simulink model "sampleModel250"  (R2021b)
settings: Solver=VariableStepAuto  StartTime=0.0  StopTime=10.0  RelTol=1e-3
undefined symbols (not defined in the file or in its folder): DiscIntNeverNeededParam, Newton, Raphson
libraries: simulink x19, slpidlib x2
settings Model: Creator=user  LastModifiedBy=user

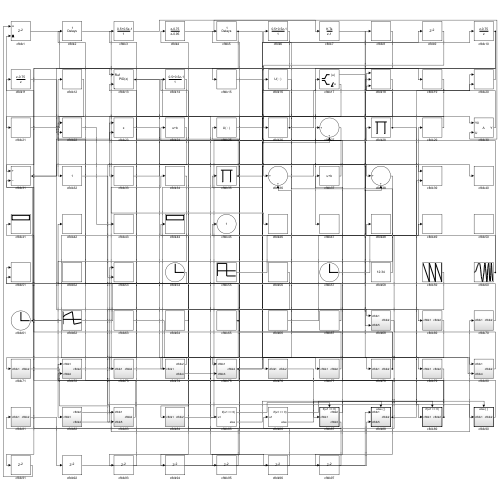
[thumbnail: Simulink's stored preview of the top-level diagram]
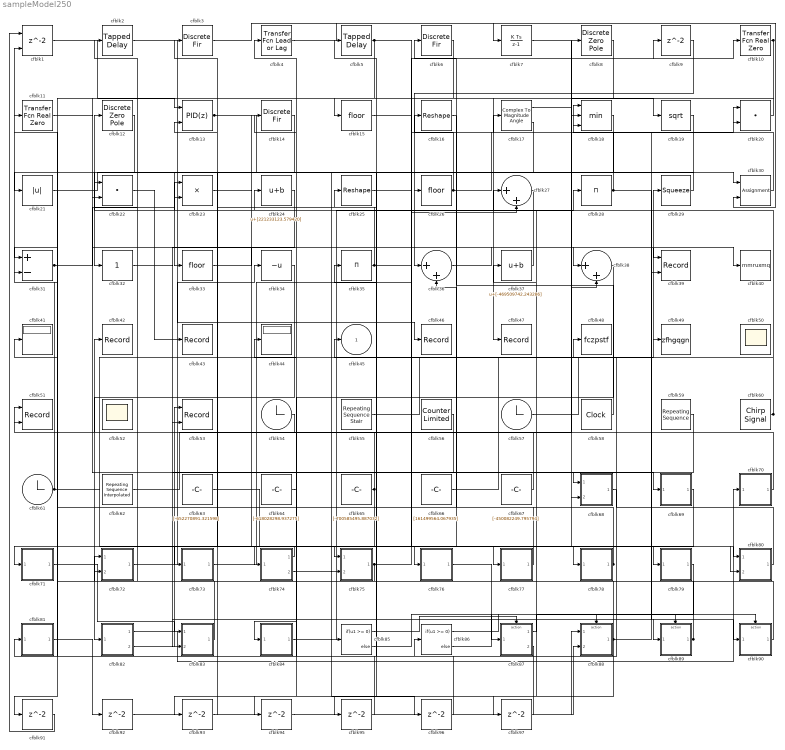
== system sampleModel250 ==
  cfblk1 : Delay  ShowEnablePort=on  SampleTime=1
      settings: InputPortMap=u0,e6
  cfblk10 : simulink/Discrete/Transfer Fcn Real Zero  ZeroZ=0.75  ICPrevInput=0.0  DoSatur=off
      settings: SourceProductBaseCode=SL
  cfblk11 : simulink/Discrete/Transfer Fcn Real Zero  ZeroZ=0.75  ICPrevInput=0.0  DoSatur=off
      settings: SourceProductBaseCode=SL
  cfblk12 : DiscreteZeroPole  Poles=[0 0.5]  Gain=1
  cfblk13 : slpidlib/PID Controller (2DOF)  Controller=PID  Form=Parallel  TimeDomain=Discrete-time  UseExternalTs=off  SampleTime=1  IntegratorMethod=Forward Euler  FilterMethod=Forward Euler  ControllerParametersSource=internal  P=1  I=1  D=0  UseFilter=on  N=100  b=1  c=1  TunerSelectOption=Transfer Function Based (PID Tuner App)  InitialConditionSource=internal  InitialConditionForIntegrator=0  InitialConditionForFilter=0  DifferentiatorICPrevScaledInput=0  ExternalReset=none  TrackingMode=off  Kt=1  LimitOutput=off  SatLimitsSource=internal  UpperSaturationLimit=inf  LowerSaturationLimit=-inf  LinearizeAsGain=off  AntiWindupMode=none  Kb=1  POutMin=[]  POutMax=[]  IOutMin=[]  IOutMax=[]  DOutMin=[]  DOutMax=[]  NOutMin=[]  NOutMax=[]  bOutMin=[]  bOutMax=[]  cOutMin=[]  cOutMax=[]  SumOutMin=[]  SumOutMax=[]  SaturationOutMin=[]  SaturationOutMax=[]  PParamMin=[]  PParamMax=[]  IParamMin=[]  IParamMax=[]  DParamMin=[]  DParamMax=[]  NParamMin=[]  NParamMax=[]  bParamMin=[]  bParamMax=[]  cParamMin=[]  cParamMax=[]  KbParamMin=[]  KbParamMax=[]  KtParamMin=[]  KtParamMax=[]  KbOutMin=[]  KbOutMax=[]  KtOutMin=[]  KtOutMax=[]  IntegratorOutMin=[]  IntegratorOutMax=[]  FilterOutMin=[]  FilterOutMax=[]  SumI1OutMin=[]  SumI1OutMax=[]  SumI2OutMin=[]  SumI2OutMax=[]  SumI3OutMin=[]  SumI3OutMax=[]  SumI4OutMin=[]  SumI4OutMax=[]  SumDOutMin=[]  SumDOutMax=[]  Sum1OutMin=[]  Sum1OutMax=[]  Sum2OutMin=[]  Sum2OutMax=[]  Sum3OutMin=[]  Sum3OutMax=[]  DifferentiatorOutMin=[]  DifferentiatorOutMax=[]  FilterDiffOutCoefMin=[]  FilterDiffOutCoefMax=[]  ReciprocalOutMin=[]  ReciprocalOutMax=[]  SumDenOutMin=[]  SumDenOutMax=[]  SumNumOutMin=[]  SumNumOutMax=[]  DivideOutMin=[]  DivideOutMax=[]  UdiffTsProdOutMin=[]  UdiffTsProdOutMax=[]  NTsProdOutMin=[]  NTsProdOutMax=[]  UintegralTsProdOutMin=[]  UintegralTsProdOutMax=[]  UngainTsProdOutMin=[]  UngainTsProdOutMax=[]  IntegratorContinuousStateAttributes=''  IntegratorStateMustResolveToSignalObject=off  IntegratorRTWStateStorageClass=Auto  FilterContinuousStateAttributes=''  FilterStateMustResolveToSignalObject=off  FilterRTWStateStorageClass=Auto  ParallelPVariant=InternalParameters  IdealPVariant=Disabled  IVariant=InternalParameters  DVariant=InternalParameters  bVariant=InternalParameters  cVariant=InternalParameters  IntegratorVariant=Discrete  SatVariant=Disabled  AWVariant=Passthrough  PCopyVariant=Disabled  TRVariant=Disabled  FdbkBlocksVariant=Forward  IdealPFdbkVariant=Disabled  SatFdbkVariant=Disabled  DerivativeFilterVariant=ForwardEulerFilter  NVariant=InternalParameters  NCopyVariant=Disabled  FilterICVariant=InternalICsFilter  IntegratorICVariant=InternalICs  ExternalResetVariant=Disabled  TRSumVariant=Passthrough  SumFdbkVariant=Disabled  SumVariant=Sum_PID  TsampFilterVariant=InternalTs  TsampNgainVariant=Passthrough  TsampIntegralVariant=Passthrough  ExternalSaturationOutDataTypeStr=Inherit: Same as second input
      settings: SourceProductBaseCode=SL
  cfblk14 : DiscreteFir  SampleTime=1
  cfblk15 : Rounding
  cfblk16 : Reshape
  cfblk17 : ComplexToMagnitudeAngle
  cfblk18 : MinMax  Inputs=3
  cfblk19 : Sqrt  SaturateOnIntegerOverflow=on
  cfblk2 : simulink/Discrete/Tapped Delay  vinit=0.0  samptime=-1  NumDelays=1  DelayOrder=Oldest  includeCurrent=off
  cfblk20 : DotProduct  InputSameDT=on  OutDataTypeStr=Inherit: Inherit via internal rule
  cfblk21 : Abs
  cfblk22 : DotProduct  InputSameDT=on  OutDataTypeStr=Inherit: Inherit via internal rule
  cfblk23 : Product
  cfblk24 : Bias  Bias=[221233123.579420]
  cfblk25 : Reshape
  cfblk26 : Rounding
  cfblk27 : Sum  Inputs=|++
  cfblk28 : Product  Inputs=*
  cfblk29 : Squeeze
  cfblk3 : DiscreteFir  SampleTime=1
  cfblk30 : Assignment  DiagnosticForDimensions=Warning  IndexOptions=Index vector (dialog)  Indices=1  OutputSizes=1
  cfblk31 : Sum  Inputs=+-
  cfblk32 : simulink/Math Operations/Slider Gain  gain=1  low=0  high=2
  cfblk33 : Rounding
  cfblk34 : UnaryMinus
  cfblk35 : Product  Inputs=*
  cfblk36 : Sum  Inputs=|++
  cfblk37 : Bias  Bias=[-469509742.243286]
  cfblk38 : Sum  Inputs=|++
  cfblk39 : Record  FileSettingsInternal="{\"entries\":[{\"content\":{\"excelSettings\":{\"content\":{},\"type\":\"Streamout.ExcelSettings\"}},\"type\":\"Streamout.FileSettingStorage\",\"uuid\":\"39295518-5782-4a04-9dda-65bbf2f7290d\"}],\"packageUris\":[\"http://schema.mathworks.com/mf0/streamout_blocks/R2020a\"],\"version\":\"1.0\"}"  Layout=[1 1]  SignalsInternal="{\"entries\":[{\"content\":{\"signals\":[{\"content\":{\"blockPath\":[\"sampleModel250/cfblk39\"],\"channel\":[],\"dimensions\":[1],\"domain\":\"sampleModel250/cfblk39\",\"lineColor\":\"#a2142f\",\"plots\":[1],\"port\":1,\"sid\":[\"\"],\"signalID\":10132,\"signalName\":\"cfblk33\"},\"type\":\"RecordBlkView.Signal\",\"uuid\":\"9efbc733-4780-4410-b863-ce1b8cd8a036\"},{\"content\":{\"blockPath\":[\"sampleModel250/cfblk39\"],\"channel\":[],\"dimensions\":[1],\"domain\":\"sampleModel250/cfblk39\",\"lineColor\":\"#139fff\",\"plots\":[1],\"port\":2,\"sid\":[\"\"],\"signalID\":10136,\"signalName\":\"cfblk61\"},\"type\":\"RecordBlkView.Signal\",\"uuid\":\"712e342f-030a-4a03-987d-c30699e0cda9\"}]},\"type\":\"RecordBlkView.InputSignals\",\"uuid\":\"45709923-ac2f-4e8a-b5ce-1ea2a88c9728\"}],\"packageUris\":[\"http://schema.mathworks.com/mf0/streamout_blocks/R2020a\"],\"version\":\"1.0\"}"  VisualizationBindings="{\"xyplotplugin\":{\"info\":[{\"series\":[{\"bindingParametersList\":[{\"parameter\":\"X-Axis\",\"signalID\":10132,\"signalName\":\"cfblk33\"},{\"parameter\":\"Y-Axis\",\"signalID\":10136,\"signalName\":\"cfblk61\"}],\"seriesID\":11867}],\"subplotID\":1}]}}"  CompatibilityTag=XY
  cfblk4 : simulink/Discrete/Transfer Fcn Lead or Lag  PoleZ=0.95  ZeroZ=0.75  ICPrevOutput=0.0  ICPrevInput=0.0  DoSatur=off
      settings: SourceProductBaseCode=SL
  cfblk40 : ToWorkspace  VariableName=mmruxmq  SaveFormat=Timeseries  SampleTime=-1
  cfblk41 : Display
  cfblk42 : Record  FileSettingsInternal="{\"entries\":[{\"content\":{\"excelSettings\":{\"content\":{},\"type\":\"Streamout.ExcelSettings\"}},\"type\":\"Streamout.FileSettingStorage\",\"uuid\":\"cb9cef44-850f-46f8-9e62-a5d9019da7f8\"}],\"packageUris\":[\"http://schema.mathworks.com/mf0/streamout_blocks/R2020a\"],\"version\":\"1.0\"}"  SignalsInternal="{\"entries\":[{\"content\":{\"signals\":[{\"content\":{\"blockPath\":[\"sampleModel250/cfblk42\"],\"channel\":[],\"dimensions\":[1],\"domain\":\"sampleModel250/cfblk42\",\"lineColor\":\"#0072bd\",\"plots\":[1],\"port\":1,\"sid\":[\"\"],\"signalID\":10168,\"signalName\":\"cfblk67\"},\"type\":\"RecordBlkView.Signal\",\"uuid\":\"09506a4d-d469-40bf-9df4-0557f256c8fa\"}]},\"type\":\"RecordBlkView.InputSignals\",\"uuid\":\"d07d11bf-0a13-4a29-ba0c-274f99fcec3c\"}],\"packageUris\":[\"http://schema.mathworks.com/mf0/streamout_blocks/R2020a\"],\"version\":\"1.0\"}"  VisualizationBindings="{\"sparklinesplugin\":{\"info\":[{\"bindingParametersList\":[],\"subplotID\":1}]}}"
  cfblk43 : Record  FileSettingsInternal="{\"entries\":[{\"content\":{\"excelSettings\":{\"content\":{},\"type\":\"Streamout.ExcelSettings\"}},\"type\":\"Streamout.FileSettingStorage\",\"uuid\":\"24f78354-d28b-420c-ba3f-fe416d6032e0\"}],\"packageUris\":[\"http://schema.mathworks.com/mf0/streamout_blocks/R2020a\"],\"version\":\"1.0\"}"  SignalsInternal="{\"entries\":[{\"content\":{\"signals\":[{\"content\":{\"blockPath\":[\"sampleModel250/cfblk43\"],\"channel\":[],\"dimensions\":[1],\"domain\":\"sampleModel250/cfblk43\",\"lineColor\":\"#139fff\",\"plots\":[1],\"port\":1,\"sid\":[\"\"],\"signalID\":10140,\"signalName\":\"cfblk22\"},\"type\":\"RecordBlkView.Signal\",\"uuid\":\"c1a6c549-0a82-4f1d-8783-18ee6ca6e206\"}]},\"type\":\"RecordBlkView.InputSignals\",\"uuid\":\"009778dc-f500-4119-a494-20fbbf5a50bc\"}],\"packageUris\":[\"http://schema.mathworks.com/mf0/streamout_blocks/R2020a\"],\"version\":\"1.0\"}"  VisualizationBindings="{\"sparklinesplugin\":{\"info\":[{\"bindingParametersList\":[],\"subplotID\":1}]}}"
  cfblk44 : Display
  cfblk46 : Record  FileSettingsInternal="{\"entries\":[{\"content\":{\"excelSettings\":{\"content\":{},\"type\":\"Streamout.ExcelSettings\"}},\"type\":\"Streamout.FileSettingStorage\",\"uuid\":\"d34b3b38-d37b-44bf-a1ca-0d6c239076fa\"}],\"packageUris\":[\"http://schema.mathworks.com/mf0/streamout_blocks/R2020a\"],\"version\":\"1.0\"}"  SignalsInternal="{\"entries\":[{\"content\":{\"signals\":[{\"content\":{\"blockPath\":[\"sampleModel250/cfblk46\"],\"channel\":[],\"dimensions\":[1],\"domain\":\"sampleModel250/cfblk46\",\"lineColor\":\"#ff6929\",\"plots\":[1],\"port\":1,\"sid\":[\"\"],\"signalID\":10144,\"signalName\":\"cfblk2\"},\"type\":\"RecordBlkView.Signal\",\"uuid\":\"5d42b0a2-1079-46c0-88f1-f1e7f1e913a3\"}]},\"type\":\"RecordBlkView.InputSignals\",\"uuid\":\"de118d10-f6e7-4dc8-9a86-7f08f8c21061\"}],\"packageUris\":[\"http://schema.mathworks.com/mf0/streamout_blocks/R2020a\"],\"version\":\"1.0\"}"  VisualizationBindings="{\"sparklinesplugin\":{\"info\":[{\"bindingParametersList\":[],\"subplotID\":1}]}}"
  cfblk47 : Record  FileSettingsInternal="{\"entries\":[{\"content\":{\"excelSettings\":{\"content\":{},\"type\":\"Streamout.ExcelSettings\"}},\"type\":\"Streamout.FileSettingStorage\",\"uuid\":\"d3a56f26-8ac3-44b7-90be-3d39ad570db3\"}],\"packageUris\":[\"http://schema.mathworks.com/mf0/streamout_blocks/R2020a\"],\"version\":\"1.0\"}"  SignalsInternal="{\"entries\":[{\"content\":{\"signals\":[{\"content\":{\"blockPath\":[\"sampleModel250/cfblk47\"],\"channel\":[],\"dimensions\":[1],\"domain\":\"sampleModel250/cfblk47\",\"lineColor\":\"#b746ff\",\"plots\":[1],\"port\":1,\"sid\":[\"\"],\"signalID\":10148,\"signalName\":\"cfblk10\"},\"type\":\"RecordBlkView.Signal\",\"uuid\":\"91dbde0a-49a0-40fd-acb2-10672f723bb8\"}]},\"type\":\"RecordBlkView.InputSignals\",\"uuid\":\"eb8da581-21b2-4b6f-8b31-33cd9e31a0d9\"}],\"packageUris\":[\"http://schema.mathworks.com/mf0/streamout_blocks/R2020a\"],\"version\":\"1.0\"}"  VisualizationBindings="{\"sparklinesplugin\":{\"info\":[{\"bindingParametersList\":[],\"subplotID\":1}]}}"
  cfblk48 : ToWorkspace  VariableName=fczpstf  SaveFormat=Timeseries  SampleTime=-1
  cfblk49 : ToWorkspace  VariableName=zfhgqgn  SaveFormat=Timeseries  SampleTime=-1
  cfblk5 : simulink/Discrete/Tapped Delay  vinit=0.0  samptime=-1  NumDelays=1  DelayOrder=Oldest  includeCurrent=off
  cfblk50 : Scope
      settings: Floating=on
  cfblk51 : Record  FileSettingsInternal="{\"entries\":[{\"content\":{\"excelSettings\":{\"content\":{},\"type\":\"Streamout.ExcelSettings\"}},\"type\":\"Streamout.FileSettingStorage\",\"uuid\":\"966ac46e-7d6c-426f-9254-bf47747501fd\"}],\"packageUris\":[\"http://schema.mathworks.com/mf0/streamout_blocks/R2020a\"],\"version\":\"1.0\"}"  Layout=[1 1]  SignalsInternal="{\"entries\":[{\"content\":{\"signals\":[{\"content\":{\"blockPath\":[\"sampleModel250/cfblk51\"],\"channel\":[],\"dimensions\":[1],\"domain\":\"sampleModel250/cfblk51\",\"lineColor\":\"#a2142f\",\"plots\":[1],\"port\":1,\"sid\":[\"\"],\"signalID\":10152,\"signalName\":\"cfblk70\"},\"type\":\"RecordBlkView.Signal\",\"uuid\":\"bcb4d5db-4b3e-4679-994d-15607dbef0df\"},{\"content\":{\"blockPath\":[\"sampleModel250/cfblk51\"],\"channel\":[],\"dimensions\":[1],\"domain\":\"sampleModel250/cfblk51\",\"lineColor\":\"#139fff\",\"plots\":[1],\"port\":2,\"sid\":[\"\"],\"signalID\":10156,\"signalName\":\"cfblk54\"},\"type\":\"RecordBlkView.Signal\",\"uuid\":\"a7bcb3c4-7ca9-4d29-a0f0-397de417030a\"}]},\"type\":\"RecordBlkView.InputSignals\",\"uuid\":\"211dfadc-f85f-49df-8759-cd0fd8e255c0\"}],\"packageUris\":[\"http://schema.mathworks.com/mf0/streamout_blocks/R2020a\"],\"version\":\"1.0\"}"  VisualizationBindings="{\"xyplotplugin\":{\"info\":[{\"series\":[{\"bindingParametersList\":[{\"parameter\":\"X-Axis\",\"signalID\":10152,\"signalName\":\"cfblk70\"},{\"parameter\":\"Y-Axis\",\"signalID\":10156,\"signalName\":\"cfblk54\"}],\"seriesID\":32821}],\"subplotID\":1}]}}"  CompatibilityTag=XY
  cfblk52 : Scope
      settings: Floating=on
  cfblk53 : Record  FileSettingsInternal="{\"entries\":[{\"content\":{\"excelSettings\":{\"content\":{},\"type\":\"Streamout.ExcelSettings\"}},\"type\":\"Streamout.FileSettingStorage\",\"uuid\":\"99a0b977-80ef-4c26-b42d-8fc2480f20f4\"}],\"packageUris\":[\"http://schema.mathworks.com/mf0/streamout_blocks/R2020a\"],\"version\":\"1.0\"}"  Layout=[1 1]  SignalsInternal="{\"entries\":[{\"content\":{\"signals\":[{\"content\":{\"blockPath\":[\"sampleModel250/cfblk53\"],\"channel\":[],\"dimensions\":[1],\"domain\":\"sampleModel250/cfblk53\",\"lineColor\":\"#a2142f\",\"plots\":[1],\"port\":1,\"sid\":[\"\"],\"signalID\":10160,\"signalName\":\"cfblk82:2\"},\"type\":\"RecordBlkView.Signal\",\"uuid\":\"1e65bc9d-8603-4a2e-9d1d-7b919e3292a0\"},{\"content\":{\"blockPath\":[\"sampleModel250/cfblk53\"],\"channel\":[],\"dimensions\":[1],\"domain\":\"sampleModel250/cfblk53\",\"lineColor\":\"#139fff\",\"plots\":[1],\"port\":2,\"sid\":[\"\"],\"signalID\":10164,\"signalName\":\"cfblk24\"},\"type\":\"RecordBlkView.Signal\",\"uuid\":\"1291a606-ac13-4bc6-a3d7-eb7377e9d85e\"}]},\"type\":\"RecordBlkView.InputSignals\",\"uuid\":\"aee4432a-cd5b-40e7-8b3a-2ad3dc5d4c9c\"}],\"packageUris\":[\"http://schema.mathworks.com/mf0/streamout_blocks/R2020a\"],\"version\":\"1.0\"}"  VisualizationBindings="{\"xyplotplugin\":{\"info\":[{\"series\":[{\"bindingParametersList\":[{\"parameter\":\"X-Axis\",\"signalID\":10160,\"signalName\":\"cfblk82:2\"},{\"parameter\":\"Y-Axis\",\"signalID\":10164,\"signalName\":\"cfblk24\"}],\"seriesID\":43266}],\"subplotID\":1}]}}"  CompatibilityTag=XY
  cfblk54 : Clock
  cfblk55 : simulink/Sources/Repeating Sequence Stair  OutValues=[579601024.933068, -400366002.756727]  tsamp=-1  OutMin=[]  OutMax=[]  OutDataTypeStr=double  OutputDataTypeScalingMode=double  OutDataType=fixdt(0,8)  ConRadixGroup=Best Precision: Vector-wise  OutScaling=2^-12
  cfblk56 : simulink/Sources/Counter Limited  uplimit=[457.000000]  tsamp=-1
  cfblk57 : Clock
  cfblk58 : DigitalClock
  cfblk59 : simulink/Sources/Repeating Sequence  rep_seq_t=[0 2]  rep_seq_y=[908061452.879816, -156366852.799595]
  cfblk6 : DiscreteFir  SampleTime=1
  cfblk60 : simulink/Sources/Chirp Signal  f1=[877541552.872540]  T=[-602399763.720180]  f2=[-816781693.848202]
  cfblk61 : Clock
  cfblk62 : simulink/Sources/Repeating Sequence Interpolated  OutValues=[233966107.012773, 455224158.955072, 827697630.012159, -499442249.113524, -329990226.707010]  TimeValues=[0 0.1 0.5 0.6 1].'  LookUpMeth=Use Input Nearest  tsamp=0.01  OutMin=[]  OutMax=[]  OutDataTypeStr=double  OutputDataTypeScalingMode=double  OutDataType=fixdt(0,8)  OutScaling=2^-10
  cfblk63 : Constant  Value=[-652270891.321598]  SampleTime=1
  cfblk64 : Constant  Value=[-618028298.937275]  SampleTime=1
  cfblk65 : Constant  Value=[-700585495.887032]  SampleTime=1
  cfblk66 : Constant  Value=[161499564.067935]  SampleTime=1
  cfblk67 : Constant  Value=[-450082249.795794]  SampleTime=1
  cfblk68 : Subsystem
  cfblk69 : Subsystem
  cfblk7 : DiscreteIntegrator  ICPrevOutput=DiscIntNeverNeededParam  ICPrevScaledInput=DiscIntNeverNeededParam
  cfblk70 : Subsystem
  cfblk71 : Subsystem
  cfblk72 : Subsystem
  cfblk73 : Subsystem
  cfblk74 : Subsystem
  cfblk75 : Subsystem
  cfblk76 : Subsystem
  cfblk77 : Subsystem
  cfblk78 : Subsystem
  cfblk79 : Subsystem
  cfblk8 : DiscreteZeroPole  Poles=[0 0.5]  Gain=1
  cfblk80 : Subsystem
  cfblk81 : Subsystem
  cfblk82 : Subsystem
  cfblk83 : Subsystem
  cfblk84 : Subsystem
  cfblk85 : If  IfExpression=u1 >= 0  SampleTime=1
  cfblk86 : If  IfExpression=u1 >= 0  SampleTime=1
  cfblk87 : Subsystem  TreatAsAtomicUnit=on
  cfblk88 : Subsystem  TreatAsAtomicUnit=on
  cfblk89 : Subsystem  TreatAsAtomicUnit=on
  cfblk{9,91..97} (8 alike) : Delay  SampleTime=1
  cfblk90 : Subsystem  TreatAsAtomicUnit=on
  cfblk45 : Outport
  wires:
  cfblk2/1 -> cfblk46/1
  cfblk10/1 -> cfblk47/1, cfblk22/2
  cfblk72/1(cfblk2) -> cfblk34/1
  cfblk22/1 -> cfblk43/1
  cfblk9/1 -> cfblk36/1
  cfblk87/1(cfblk2) -> cfblk37/1
  cfblk68/1(cfblk2) -> cfblk86/1
  cfblk19/1 -> cfblk32/1
  cfblk82/1(cfblk2) -> cfblk70/1(cfblk1)
  cfblk29/1 -> cfblk26/1
  cfblk84/1(cfblk2) -> cfblk28/1
  cfblk37/1 -> cfblk12/1
  cfblk63/1 -> cfblk77/1(cfblk1)
  cfblk20/1 -> cfblk15/1
  cfblk82/2(cfblk4) -> cfblk53/1
  cfblk87/2(cfblk3) -> cfblk81/1(cfblk1)
  cfblk57/1 -> cfblk29/1
  cfblk14/1 -> cfblk33/1
  cfblk35/1 -> cfblk79/1(cfblk1), cfblk3/1
  cfblk73/1(cfblk2) -> cfblk10/1
  cfblk30/1 -> cfblk18/1
  cfblk31/1 -> cfblk23/1, cfblk38/1
  cfblk74/1(cfblk2) -> cfblk71/1(cfblk1)
  cfblk1/1 -> cfblk13/1
  cfblk62/1 -> cfblk8/1
  cfblk7/1 -> cfblk19/1
  cfblk36/1 -> cfblk40/1
  cfblk71/1(cfblk2) -> cfblk83/1(cfblk1)
  cfblk70/1(cfblk2) -> cfblk51/1
  cfblk21/1 -> cfblk30/1
  cfblk4/1 -> cfblk30/2
  cfblk88/1(cfblk2) -> cfblk27/1, cfblk25/1, cfblk20/2, cfblk93/1
  cfblk61/1 -> cfblk1/2, cfblk39/2, cfblk80/2(cfblk4)
  cfblk69/1(cfblk2) -> cfblk74/1(cfblk1)
  cfblk32/1 -> cfblk89/1(cfblk1)
  cfblk58/1 -> cfblk6/1
  cfblk78/1(cfblk2) -> cfblk41/1, cfblk5/1
  cfblk60/1 -> cfblk24/1, cfblk45/1
  cfblk34/1 -> cfblk82/1(cfblk1)
  cfblk89/1(cfblk2) -> cfblk44/1, cfblk22/1
  cfblk28/1 -> cfblk90/1(cfblk1), cfblk18/3
  cfblk55/1 -> cfblk18/2
  cfblk27/1 -> cfblk23/2
  cfblk26/1 -> cfblk16/1, cfblk20/1
  cfblk77/1(cfblk2) -> cfblk36/2
  cfblk15/1 -> cfblk68/1(cfblk1)
  cfblk66/1 -> cfblk49/1
  cfblk3/1 -> cfblk7/1
  cfblk56/1 -> cfblk83/2(cfblk5)
  cfblk24/1 -> cfblk53/2
  cfblk13/1 -> cfblk85/1, cfblk38/2
  cfblk17/1 -> cfblk80/1(cfblk1)
  cfblk16/1 -> cfblk76/1(cfblk1)
  cfblk5/1 -> cfblk31/1, cfblk27/2
  cfblk80/1(cfblk2) -> cfblk48/1
  cfblk11/1 -> cfblk69/1(cfblk1)
  cfblk67/1 -> cfblk42/1
  cfblk17/2 -> cfblk73/1(cfblk1)
  cfblk8/1 -> cfblk68/2(cfblk5)
  cfblk33/1 -> cfblk39/1
  cfblk83/1(cfblk2) -> cfblk31/2
  cfblk65/1 -> cfblk2/1, cfblk75/2(cfblk3)
  cfblk59/1 -> cfblk84/1(cfblk1)
  cfblk6/1 -> cfblk21/1
  cfblk23/1 -> cfblk75/1(cfblk1)
  cfblk75/1(cfblk2) -> cfblk9/1, cfblk72/2(cfblk4), cfblk17/1
  cfblk54/1 -> cfblk51/2
  cfblk64/1 -> cfblk14/1
  cfblk90/1(cfblk2) -> cfblk72/1(cfblk1)
  cfblk25/1 -> cfblk78/1(cfblk1)
  cfblk76/1(cfblk2) -> cfblk87/1(cfblk1)
  cfblk85/1 -> cfblk87/Action
  cfblk85/2 -> cfblk88/Action
  cfblk86/1 -> cfblk89/Action
  cfblk86/2 -> cfblk90/Action
  cfblk12/1 -> cfblk91/1
  cfblk91/1 -> cfblk1/1
  cfblk81/1(cfblk2) -> cfblk92/1
  cfblk92/1 -> cfblk88/1(cfblk1)
  cfblk93/1 -> cfblk13/2
  cfblk38/1 -> cfblk94/1
  cfblk94/1 -> cfblk88/2(cfblk5)
  cfblk18/1 -> cfblk95/1
  cfblk95/1 -> cfblk4/1
  cfblk74/2(cfblk4) -> cfblk96/1
  cfblk96/1 -> cfblk11/1
  cfblk79/1(cfblk2) -> cfblk97/1
  cfblk97/1 -> cfblk35/1

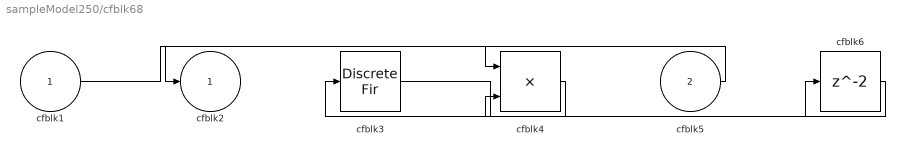
== system sampleModel250/cfblk68 ==
  cfblk1 : Inport
  cfblk5 : Inport  Port=2
  cfblk3 : DiscreteFir  SampleTime=1
  cfblk4 : Product  Inputs=**
  cfblk6 : Delay  SampleTime=1
  cfblk2 : Outport
  wires:
  cfblk5/1 -> cfblk2/1
  cfblk4/1 -> cfblk3/1
  cfblk1/1 -> cfblk4/1
  cfblk3/1 -> cfblk6/1
  cfblk6/1 -> cfblk4/2

== system sampleModel250/cfblk69 ==
  cfblk1 : Inport
  cfblk3 : simulink/Discrete/Tapped Delay  vinit=0.0  samptime=-1  NumDelays=1  DelayOrder=Oldest  includeCurrent=off
  cfblk2 : Outport
  wires:
  cfblk1/1 -> cfblk3/1
  cfblk3/1 -> cfblk2/1

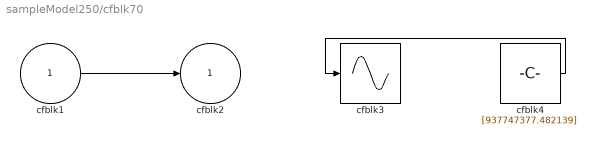
== system sampleModel250/cfblk70 ==
  cfblk1 : Inport
  cfblk3 : Sin  TimeSource=Use external signal  SampleTime=0
  cfblk4 : Constant  Value=[937747377.482139]  SampleTime=1
  cfblk2 : Outport
  wires:
  cfblk1/1 -> cfblk2/1
  cfblk4/1 -> cfblk3/1

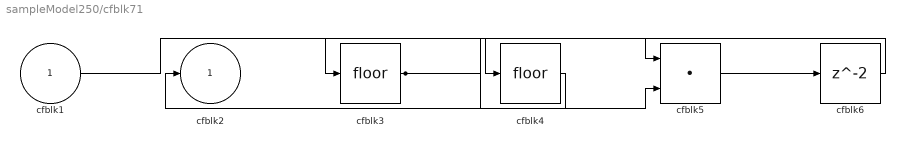
== system sampleModel250/cfblk71 ==
  cfblk1 : Inport
  cfblk3 : Rounding
  cfblk4 : Rounding
  cfblk5 : DotProduct  InputSameDT=on  OutDataTypeStr=Inherit: Inherit via internal rule
  cfblk6 : Delay  SampleTime=1
  cfblk2 : Outport
  wires:
  cfblk4/1 -> cfblk2/1
  cfblk1/1 -> cfblk4/1
  cfblk3/1 -> cfblk5/1, cfblk5/2
  cfblk5/1 -> cfblk6/1
  cfblk6/1 -> cfblk3/1

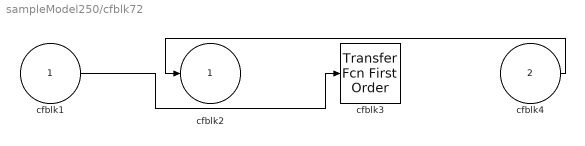
== system sampleModel250/cfblk72 ==
  cfblk1 : Inport
  cfblk4 : Inport  Port=2
  cfblk3 : simulink/Discrete/Transfer Fcn First Order  PoleZ=0.95  ICPrevOutput=0.0  DoSatur=off
  cfblk2 : Outport
  wires:
  cfblk4/1 -> cfblk2/1
  cfblk1/1 -> cfblk3/1

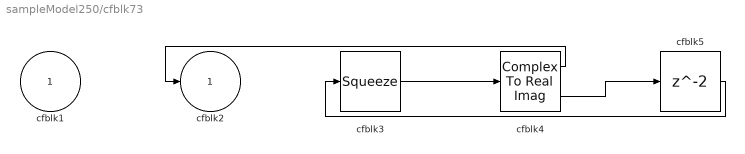
== system sampleModel250/cfblk73 ==
  cfblk1 : Inport
  cfblk3 : Squeeze
  cfblk4 : ComplexToRealImag
  cfblk5 : Delay  SampleTime=1
  cfblk2 : Outport
  wires:
  cfblk4/1 -> cfblk2/1
  cfblk3/1 -> cfblk4/1
  cfblk4/2 -> cfblk5/1
  cfblk5/1 -> cfblk3/1

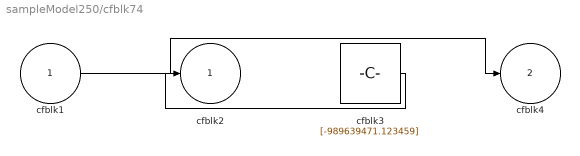
== system sampleModel250/cfblk74 ==
  cfblk1 : Inport
  cfblk3 : Constant  Value=[-989639471.123459]  SampleTime=1
  cfblk2 : Outport
  cfblk4 : Outport  Port=2
  wires:
  cfblk1/1 -> cfblk4/1
  cfblk3/1 -> cfblk2/1

== system sampleModel250/cfblk75 ==
  cfblk1 : Inport
  cfblk3 : Inport  Port=2
  cfblk2 : Outport
  wires:
  cfblk3/1 -> cfblk2/1

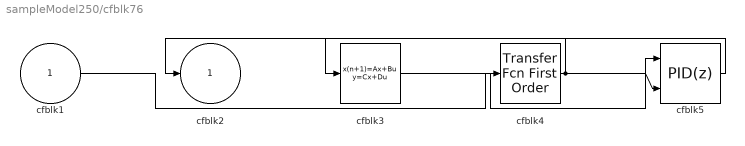
== system sampleModel250/cfblk76 ==
  cfblk1 : Inport
  cfblk3 : DiscreteStateSpace
  cfblk4 : simulink/Discrete/Transfer Fcn First Order  PoleZ=0.95  ICPrevOutput=0.0  DoSatur=off
  cfblk5 : slpidlib/PID Controller (2DOF)  Controller=PID  Form=Parallel  TimeDomain=Discrete-time  UseExternalTs=off  SampleTime=1  IntegratorMethod=Forward Euler  FilterMethod=Forward Euler  ControllerParametersSource=internal  P=1  I=1  D=0  UseFilter=on  N=100  b=1  c=1  TunerSelectOption=Transfer Function Based (PID Tuner App)  InitialConditionSource=internal  InitialConditionForIntegrator=0  InitialConditionForFilter=0  DifferentiatorICPrevScaledInput=0  ExternalReset=none  TrackingMode=off  Kt=1  LimitOutput=off  SatLimitsSource=internal  UpperSaturationLimit=inf  LowerSaturationLimit=-inf  LinearizeAsGain=off  AntiWindupMode=none  Kb=1  POutMin=[]  POutMax=[]  IOutMin=[]  IOutMax=[]  DOutMin=[]  DOutMax=[]  NOutMin=[]  NOutMax=[]  bOutMin=[]  bOutMax=[]  cOutMin=[]  cOutMax=[]  SumOutMin=[]  SumOutMax=[]  SaturationOutMin=[]  SaturationOutMax=[]  PParamMin=[]  PParamMax=[]  IParamMin=[]  IParamMax=[]  DParamMin=[]  DParamMax=[]  NParamMin=[]  NParamMax=[]  bParamMin=[]  bParamMax=[]  cParamMin=[]  cParamMax=[]  KbParamMin=[]  KbParamMax=[]  KtParamMin=[]  KtParamMax=[]  KbOutMin=[]  KbOutMax=[]  KtOutMin=[]  KtOutMax=[]  IntegratorOutMin=[]  IntegratorOutMax=[]  FilterOutMin=[]  FilterOutMax=[]  SumI1OutMin=[]  SumI1OutMax=[]  SumI2OutMin=[]  SumI2OutMax=[]  SumI3OutMin=[]  SumI3OutMax=[]  SumI4OutMin=[]  SumI4OutMax=[]  SumDOutMin=[]  SumDOutMax=[]  Sum1OutMin=[]  Sum1OutMax=[]  Sum2OutMin=[]  Sum2OutMax=[]  Sum3OutMin=[]  Sum3OutMax=[]  DifferentiatorOutMin=[]  DifferentiatorOutMax=[]  FilterDiffOutCoefMin=[]  FilterDiffOutCoefMax=[]  ReciprocalOutMin=[]  ReciprocalOutMax=[]  SumDenOutMin=[]  SumDenOutMax=[]  SumNumOutMin=[]  SumNumOutMax=[]  DivideOutMin=[]  DivideOutMax=[]  UdiffTsProdOutMin=[]  UdiffTsProdOutMax=[]  NTsProdOutMin=[]  NTsProdOutMax=[]  UintegralTsProdOutMin=[]  UintegralTsProdOutMax=[]  UngainTsProdOutMin=[]  UngainTsProdOutMax=[]  IntegratorContinuousStateAttributes=''  IntegratorStateMustResolveToSignalObject=off  IntegratorRTWStateStorageClass=Auto  FilterContinuousStateAttributes=''  FilterStateMustResolveToSignalObject=off  FilterRTWStateStorageClass=Auto  ParallelPVariant=InternalParameters  IdealPVariant=Disabled  IVariant=InternalParameters  DVariant=InternalParameters  bVariant=InternalParameters  cVariant=InternalParameters  IntegratorVariant=Discrete  SatVariant=Disabled  AWVariant=Passthrough  PCopyVariant=Disabled  TRVariant=Disabled  FdbkBlocksVariant=Forward  IdealPFdbkVariant=Disabled  SatFdbkVariant=Disabled  DerivativeFilterVariant=ForwardEulerFilter  NVariant=InternalParameters  NCopyVariant=Disabled  FilterICVariant=InternalICsFilter  IntegratorICVariant=InternalICs  ExternalResetVariant=Disabled  TRSumVariant=Passthrough  SumFdbkVariant=Disabled  SumVariant=Sum_PID  TsampFilterVariant=InternalTs  TsampNgainVariant=Passthrough  TsampIntegralVariant=Passthrough  ExternalSaturationOutDataTypeStr=Inherit: Same as second input
      settings: SourceProductBaseCode=SL
  cfblk2 : Outport
  wires:
  cfblk5/1 -> cfblk2/1
  cfblk3/1 -> cfblk5/1
  cfblk1/1 -> cfblk4/1
  cfblk4/1 -> cfblk5/2, cfblk3/1

== system sampleModel250/cfblk77 ==
  cfblk1 : Inport
  cfblk3 : Trigonometry
  cfblk2 : Outport
  wires:
  cfblk1/1 -> cfblk3/1
  cfblk3/1 -> cfblk2/1

== system sampleModel250/cfblk78 ==
  cfblk1 : Inport
  cfblk3 : Sqrt  Operator=rSqrt  AlgorithmType=Newton-Raphson  SaturateOnIntegerOverflow=on
  cfblk2 : Outport
  wires:
  cfblk1/1 -> cfblk3/1
  cfblk3/1 -> cfblk2/1

== system sampleModel250/cfblk79 ==
  cfblk1 : Inport
  cfblk3 : simulink/Math Operations/Slider Gain  gain=1  low=0  high=2
  cfblk2 : Outport
  wires:
  cfblk3/1 -> cfblk2/1
  cfblk1/1 -> cfblk3/1

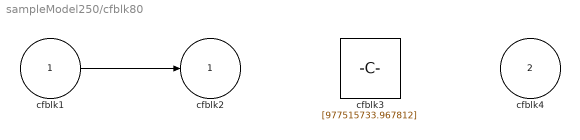
== system sampleModel250/cfblk80 ==
  cfblk1 : Inport
  cfblk4 : Inport  Port=2
  cfblk3 : Constant  Value=[977515733.967812]  SampleTime=1
  cfblk2 : Outport
  wires:
  cfblk1/1 -> cfblk2/1

== system sampleModel250/cfblk81 ==
  cfblk1 : Inport
  cfblk3 : Polyval  Coefs=[ +2.081618890e-019, -1.441693666e-014, +4.719686976e-010, -8.536869453e-006, +1.621573104e-001, -8.087801117e+001 ]
  cfblk4 : Signum
  cfblk2 : Outport
  wires:
  cfblk1/1 -> cfblk4/1
  cfblk4/1 -> cfblk3/1
  cfblk3/1 -> cfblk2/1

== system sampleModel250/cfblk82 ==
  cfblk1 : Inport
  cfblk3 : Polyval  Coefs=[ +2.081618890e-019, -1.441693666e-014, +4.719686976e-010, -8.536869453e-006, +1.621573104e-001, -8.087801117e+001 ]
  cfblk2 : Outport
  cfblk4 : Outport  Port=2
  wires:
  cfblk1/1 -> cfblk3/1, cfblk2/1
  cfblk3/1 -> cfblk4/1

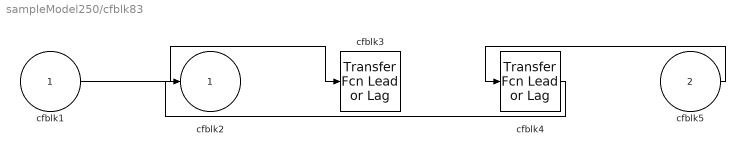
== system sampleModel250/cfblk83 ==
  cfblk1 : Inport
  cfblk5 : Inport  Port=2
  cfblk3 : simulink/Discrete/Transfer Fcn Lead or Lag  PoleZ=0.95  ZeroZ=0.75  ICPrevOutput=0.0  ICPrevInput=0.0  DoSatur=off
      settings: SourceProductBaseCode=SL
  cfblk4 : simulink/Discrete/Transfer Fcn Lead or Lag  PoleZ=0.95  ZeroZ=0.75  ICPrevOutput=0.0  ICPrevInput=0.0  DoSatur=off
      settings: SourceProductBaseCode=SL
  cfblk2 : Outport
  wires:
  cfblk5/1 -> cfblk4/1
  cfblk1/1 -> cfblk3/1
  cfblk4/1 -> cfblk2/1

== system sampleModel250/cfblk84 ==
  cfblk1 : Inport
  cfblk3 : simulink/Discrete/Difference  ICPrevInput=0.0  OutMin=[]  OutMax=[]  OutDataTypeStr=Inherit: Inherit via back propagation  OutDataType=fixdt(1, 16)  OutScaling=2^-10  DoSatur=off
  cfblk4 : Constant  Value=[-822256036.617830]  SampleTime=1
  cfblk2 : Outport
  wires:
  cfblk4/1 -> cfblk3/1
  cfblk1/1 -> cfblk2/1

== system sampleModel250/cfblk87 ==
  cfblk1 : Inport
  Action Port : ActionPort  ActionPortLabel=if(u1 >= 0)
  cfblk2 : Outport
  cfblk3 : Outport  Port=2
  wires:
  cfblk1/1 -> cfblk2/1, cfblk3/1

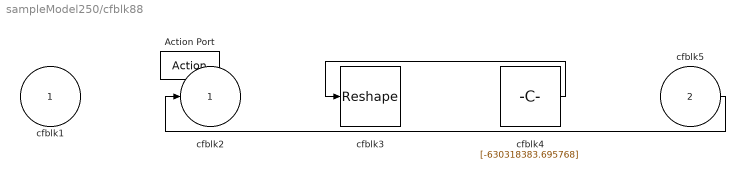
== system sampleModel250/cfblk88 ==
  cfblk1 : Inport
  cfblk5 : Inport  Port=2
  Action Port : ActionPort  ActionPortLabel=else
  cfblk3 : Reshape
  cfblk4 : Constant  Value=[-630318383.695768]  SampleTime=1
  cfblk2 : Outport
  wires:
  cfblk5/1 -> cfblk2/1
  cfblk4/1 -> cfblk3/1

== system sampleModel250/cfblk89 ==
  cfblk1 : Inport
  Action Port : ActionPort  ActionPortLabel=if(u1 >= 0)
  cfblk3 : simulink/Discrete/Difference  ICPrevInput=0.0  OutMin=[]  OutMax=[]  OutDataTypeStr=Inherit: Inherit via back propagation  OutDataType=fixdt(1, 16)  OutScaling=2^-10  DoSatur=off
  cfblk2 : Outport
  wires:
  cfblk1/1 -> cfblk3/1
  cfblk3/1 -> cfblk2/1

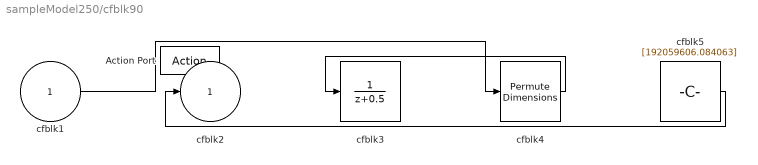
== system sampleModel250/cfblk90 ==
  cfblk1 : Inport
  Action Port : ActionPort  ActionPortLabel=else
  cfblk3 : DiscreteTransferFcn
  cfblk4 : PermuteDimensions
  cfblk5 : Constant  Value=[192059606.084063]  SampleTime=1
  cfblk2 : Outport
  wires:
  cfblk5/1 -> cfblk2/1
  cfblk1/1 -> cfblk4/1
  cfblk4/1 -> cfblk3/1
